simulink model "determineIterationPhase_th"  (R2018a)
settings: Solver=FixedStepAuto  StartTime=0.0  StopTime=100  FixedStep=sm.Ts  RelTol=1e-3
libraries: determineIterationPhase_ul x1
settings Model: Creator=mitch  LastModifiedBy=mitch

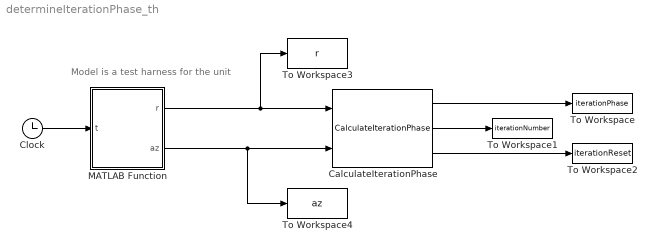
== system determineIterationPhase_th ==
  note: Model is a test harness for the unit
  CalculateIterationPhase : determineIterationPhase_ul/CalculateIterationPhase
  Clock : Clock
  MATLAB Function : MATLAB Function  TreatAsAtomicUnit=on
  To Workspace : ToWorkspace  VariableName=iterationPhase  SaveFormat=Timeseries  SampleTime=-1
  To Workspace1 : ToWorkspace  VariableName=iterationNumber  SaveFormat=Timeseries  SampleTime=-1
  To Workspace2 : ToWorkspace  VariableName=iterationReset  SaveFormat=Timeseries  SampleTime=-1
  To Workspace3 : ToWorkspace  VariableName=r  SaveFormat=Timeseries  SampleTime=-1
  To Workspace4 : ToWorkspace  VariableName=az  SaveFormat=Timeseries  SampleTime=-1
  wires:
  Clock/1 -> MATLAB Function/1(t)
  MATLAB Function/1(r) -> To Workspace3/1, CalculateIterationPhase/1
  CalculateIterationPhase/1 -> To Workspace/1
  CalculateIterationPhase/2 -> To Workspace1/1
  CalculateIterationPhase/3 -> To Workspace2/1
  MATLAB Function/2(az) -> To Workspace4/1, CalculateIterationPhase/2

== matlab function determineIterationPhase_th/MATLAB Function ==
  data: t input; r output; az output
function [r,az] = fcn(t)

r = 70+35*sin(2*pi*t/20);
az = cos(2*pi*t/20);

end
